simulink model "chapt5_MPC_Dynamics_AFS"  (Simulink 8.2)
settings: Solver=ode45  StartTime=0.0  StopTime=20  FixedStep=0.01  RelTol=1e-3
libraries: Solver_SF x1
settings Model: Creator=xuwei  LastModifiedBy=leoking99

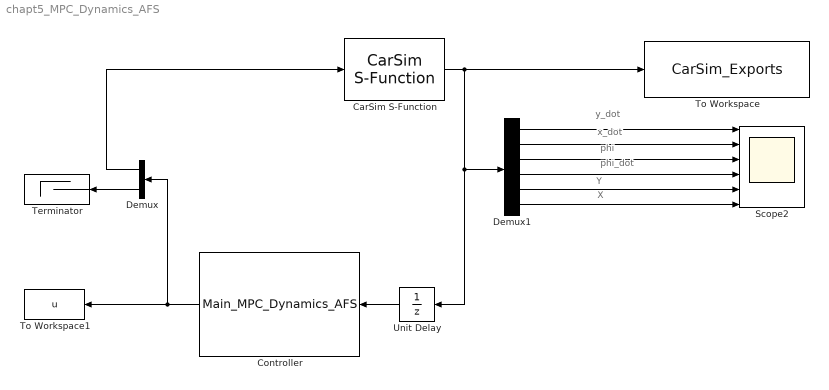
== system chapt5_MPC_Dynamics_AFS ==
  note: y_dot
  note: x_dot
  note: phi
  note: phi_dot
  note: Y
  note: X
  CarSim S-Function : Solver_SF/CarSim S-Function  Priority=1  VehicleCode=i_s  SIMFILE=chapt5_Dynamics_AFS.sim
  Controller : S-Function  FunctionName=Main_MPC_Dynamics_AFS  EnableBusSupport=off
  Demux : Demux  Outputs=[1, 6]
  Demux1 : Demux  Outputs=6
  Scope2 : Scope  NumInputPorts=6
      settings: TimeRange=20  YMin=-1~35~-10~-20~-4~0  YMax=1~36.5~5~20~2~200
  Terminator : Terminator
  To Workspace : ToWorkspace  VariableName=CarSim_Exports  SampleTime=-1  SaveFormat=Structure
  To Workspace1 : ToWorkspace  VariableName=u  SampleTime=-1  SaveFormat=Structure
  Unit Delay : UnitDelay  SampleTime=-1
  wires:
  CarSim S-Function/1 -> Unit Delay/1, Demux1/1, To Workspace/1
  Demux1/1 -> Scope2/1
  Demux1/2 -> Scope2/2
  Demux1/3 -> Scope2/3
  Demux1/4 -> Scope2/4
  Demux1/5 -> Scope2/5
  Demux1/6 -> Scope2/6
  Unit Delay/1 -> Controller/1
  Controller/1 -> Demux/1, To Workspace1/1
  Demux/1 -> CarSim S-Function/1
  Demux/2 -> Terminator/1
